simulink library "lib_Convection_TurbFlatPlatePowLawTempVary"  (R2015a)
settings: Solver=ode45  StartTime=0.0  StopTime=10.0  RelTol=1e-3
settings Model: Creator=jlkratz  LastModifiedBy=jlkratz

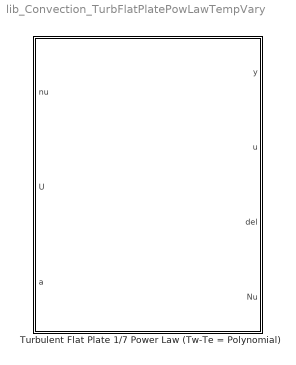
== system lib_Convection_TurbFlatPlatePowLawTempVary ==
  Turbulent Flat Plate 1/7 Power Law (Tw-Te = Polynomial) : Subsystem  mask(TSAT: Turbulent Flat Plate 1/7 Power Law (Tw-Te = Polynomial)){Pr_M=1, x_M=[0.05:0.05:5], n_M=50, BN_M=double(gcb)}
      mask prompts: Pr_M "Pr_M - Prandtl number"; x_M "x_M - Locations along the surface to compute the boundary layer for [mx1]"; n_M "n_M - Number of elements in the boundary layer"; BN_M "BN_M - Block name"
      mask help:
      | The block employs the 1/7 Power Law for incompressible turbulent flow over a flat plat with varying wall temperature (Tw) and or free-stream temperature (Te). The variation in temperature is assumed to be represented by a polynomial:
      |
      | Tw - Te = a0 + a1*x + a2*x^2 + ... + aN*x^N
      |
      | The 1/7 Power Law assumes the mean velocity (u) in the boundary layer and wall temperature minus the mean temperature (T) in the boundary layer vary with y^(1/7) where y is the distance from the surface of the wall. Temperature variations are accounted for using the method of indicial solutions based on the principle of superposition which is applicable give the thermal-energy equation is linear.
      |
      | See the block help menu for more details.
      mask init:
      | %Error/Warning Checking --------------------------------------------------%
      | 
      | %---- Pr_M ----%
      | %Scalar?
      | if isscalar(Pr_M) == 0
      |     Pr_M = 1;
      |     fprintf('Warning in %s: Pr_M must be a scalar. Pr_M has been set equal to 1 for computations.\n',char(BN_M));
      | end
      | %Real?
      | if isreal(Pr_M) == 0
      |     Pr_M = real(Pr_M);
      |     fprintf('Warning in %s: Pr_M must be a real. Pr_M has been set equal to real part of the entered value for computations.\n',char(BN_M));
      | end
      | %Finite?
      | if isfinite(Pr_M) == 0
      |     Pr_M = 1;
      |     fprintf('Warning in %s: Pr_M must be a finite. Pr_M has been set equal to 1 for computations.\n',char(BN_M));
      | end
      | %greater than 0
      | if Pr_M <= 0
      |     Pr_M = 0.01;
      |     fprintf('Warning in %s: Pr_M must be positive. Pr_M has been set equal to 0.01 for computations.\n',char(BN_M));
      | end
      | %Between 0.01 and 40000
      | if Pr_M < 0.01 || Pr_M > 40000
      |     fprintf('Warning in %s: Pr_M is outside of recommended range of Prandtl numbers (0.01 < Pr < 40000). Results could be erroneous.\n',char(BN_M));
      | end
      | %---- x_M ----%
      | %Not empty?
      | if isempty(x_M) == 1
      |     x_M = [0.1 0.5 1];
      |     fprintf('Warning in %s: x_M cannot be empty. x_M has been set to [0.1 0.5 1] for computations.\n',char(BN_M));
      | end
      | %1-D array?
      | if min(size(x_M)) ~= 1 || length(size(x_M)) > 2
      |     x_M = [0.1 0.5 1];
      |     fprintf('Warning in %s: x_M must be a 1-D array. x_M has been set to [0.1 0.5 1] for computations.\n',char(BN_M));
      | end
      | %Real?
      | if min(isreal(x_M)) == 0
      |     x_M = real(x_M);
      |     fprintf('Warning in %s: x_M must have all real elements. x_M has been set equal to the real parts of the entered values for computations.\n',char(BN_M));
      | end
      | %Finite?
      | if min(isfinite(x_M)) == 0
      |     x_M = [0.1 0.5 1];
      |     fprintf('Warning in %s: x_M must have all finite elements. x_M has been set equal to [0.1 0.5 1] for computations.\n',char(BN_M));
      | end
      | %Greater than 0?
      | if min(x_M) <= 0
      |     x_M = [0.1 0.5 1];
      |     fprintf('Warning in %s: x_M must have all elements that are greater than 0. x_M has been set equal to [0.1 0.5 1] for computations.\n',char(BN_M));
      | end
      | %Monotonically Increasing?
      | if max(size(x_M)) > 1
      |     if min(diff(x_M)) <= 0
      |         x_M = unique(sort(x_M));
      |         fprintf('Warning in %s: x_M must be a monotonically increasing array. x_M has been put in ascending order with redundant elements removed for computations\n',char(BN_M));
      |     end
      | end
      | %---- n_M ----%
      | %Scalar?
      | if isscalar(n_M) == 0
      |     n_M = 10;
      |     fprintf('Warning in %s: n_M must be a scalar. n_M has been set equal to 10 for computations.\n',char(BN_M));
      | end
      | %Real?
      | if isreal(n_M) == 0
      |     n_M = real(n_M);
      |     fprintf('Warning in %s: n_M must be a real. n_M has been set equal to real part of the entered value for computations.\n',char(BN_M));
      | end
      | %Finite?
      | if isfinite(n_M) == 0
      |     n_M = 10;
      |     fprintf('Warning in %s: n_M must be a finite. n_M has been set equal to 10 for computations.\n',char(BN_M));
      | end
      | %Integer?
      | if rem(n_M,1) > 0
      |     n_M = round(n_M);
      |     fprintf('Warning in %s: n_M must be an integer. n_M has been rounded to the closest integer.\n',char(BN_M));
      | end
      | %Greater than 1?
      | if n_M <= 1
      |     n_M = 2;
      |     fprintf('Warning in %s: n_M must be 2 or greater. n_M has been set equal to 2 for computations.\n',char(BN_M));
      | end
      mask Help: web(which('Convection_TSAT_TurbBLPowerLawTempVary.html'),'-helpbrowser')

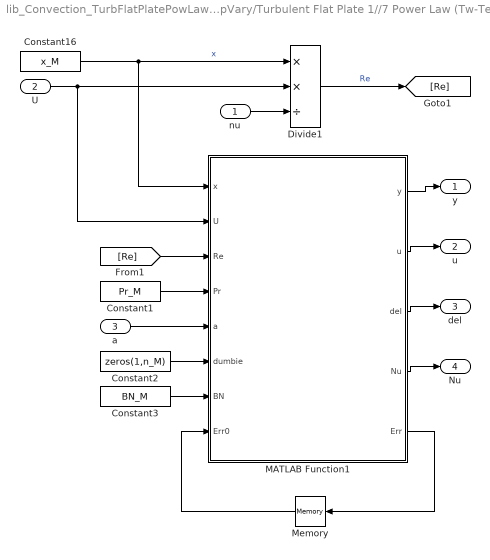
== system lib_Convection_TurbFlatPlatePowLawTempVary/Turbulent Flat Plate 1//7 Power Law (Tw-Te = Polynomial) ==
  nu : Inport
  U : Inport  Port=2
  a : Inport  Port=3
  Constant1 : Constant  Value=Pr_M
  Constant16 : Constant  Value=x_M
  Constant2 : Constant  Value=zeros(1,n_M)
  Constant3 : Constant  Value=BN_M
  Divide1 : Product  Inputs=**/
  MATLAB Function1 : MATLAB Function  TreatAsAtomicUnit=on
  Memory : Memory  X0=zeros(1,14)
  y : Outport
  u : Outport  Port=2
  del : Outport  Port=3
  Nu : Outport  Port=4
  wires:
  Constant2/1 -> MATLAB Function1/6(dumbie)
  Constant1/1 -> MATLAB Function1/4(Pr)
  U/1 -> Divide1/2, MATLAB Function1/2(U)
  a/1 -> MATLAB Function1/5(a)
  [Re] -> MATLAB Function1/3(Re)
  MATLAB Function1/3(del) -> del/1
  MATLAB Function1/4(Nu) -> Nu/1
  MATLAB Function1/1(y) -> y/1
  MATLAB Function1/2(u) -> u/1
  nu/1 -> Divide1/3
  Constant16/1 -> Divide1/1, MATLAB Function1/1(x)  "x"
  Divide1/1 -> [Re]  "Re"
  MATLAB Function1/5(Err) -> Memory/1
  Memory/1 -> MATLAB Function1/8(Err0)
  Constant3/1 -> MATLAB Function1/7(BN)

== matlab function lib_Convection_TurbFlatPlatePowLawTempVary/Turbulent Flat Plate 1//7 Power Law (Tw-Te = Polynomial)/MATLAB Function1 ==
  data: x input; U input; Re input; Pr input; a input; y output; u output; dumbie input; BN input; del output; Nu output; Err0 input; Err output
function [y, u, del, Nu, Err] = BoundaryLayerCalcs(x,U,Re,Pr,a,dumbie,BN,Err0)
%#codegen

%Description
% This function block computes dimensional quantities and forms the outputs

%Inputs:
% x - spatial variable along the surface [mx1]
% U - free-stream velocity [mx1]
% Re - Reynolds number [mx1]
% Pr - Prandtl number [1x1]
% a - array with polynomial coefficients for Tw-Te [px1]

%Outputs:
% y - dimensional y-coordinates for the velocity profile [nxm]
% U - velocity profile U(x,y) [nxm]
% del - hydrodynamic boundary layer thickness, del(x) [mx1]
% Nu - Nusselt number, Nu(x)[mx1]

%Error/Warning Checks ----------------------------------------------------%

Err = Err0;
ErrNum = 1;
%---- Re ----%
%Not empty?
if isempty(Re) == 1 &&  Err(ErrNum) == 0
    Err(ErrNum) = 1;
    fprintf('Warning in %s: Re is an empty array. It is suggested you check nu and x_M for sources of the error.\n',char(BN));
end
ErrNum = ErrNum + 1;
%1D array the length of x?
if (min(size(Re)) > 1 || length(size(Re)) > 2) && Err(ErrNum) == 0
    Err(ErrNum) = 1;
    fprintf('Warning in %s: Re must be a 1-D array. It is suggested you check nu and x_M for sources of the error.\n',char(BN));
end
ErrNum = ErrNum + 1;
%Real?
if min(isreal(Re)) < 1 && Err(ErrNum) == 0
    Err(ErrNum) = 1;
    fprintf('Warning in %s: Re must have all real elements. It is suggested you check nu and x_M for sources of the error.\n',char(BN));
end
ErrNum = ErrNum + 1;
%Finite?
if min(isfinite(Re)) < 1 && Err(ErrNum) == 0
    Err(ErrNum) = 1;
    fprintf('Warning in %s: Re must have all finite elements. It is suggested you check nu and x_M for sources of the error.\n',char(BN));
end
ErrNum = ErrNum + 1;
%Positive?
if min(Re) <= 0 && Err(ErrNum) == 0
    Err(ErrNum) = 1;
    fprintf('Warning in %s: Re must be great than 0. It is suggested you check nu and x_M for sources of the error.\n',char(BN));
end
ErrNum = ErrNum + 1;
%---- U ----%
%Not empty?
if isempty(U) == 1 &&  Err(ErrNum) == 0
    Err(ErrNum) = 1;
    fprintf('Warning in %s: U is an empty array.\n',char(BN));
end
ErrNum = ErrNum + 1;
%1D array the length of x?
if (min(size(U)) > 1 || length(size(U)) > 2) && Err(ErrNum) == 0
    Err(ErrNum) = 1;
    fprintf('Warning in %s: U must be a 1-D array.\n',char(BN));
end
ErrNum = ErrNum + 1;
%Real?
if min(isreal(U)) < 1 && Err(ErrNum) == 0
    Err(ErrNum) = 1;
    fprintf('Warning in %s: U must have all real elements.\n',char(BN));
end
ErrNum = ErrNum + 1;
%Finite?
if min(isfinite(U)) < 1 && Err(ErrNum) == 0
    Err(ErrNum) = 1;
    fprintf('Warning in %s: U must have all finite elements.\n',char(BN));
end
ErrNum = ErrNum + 1;
%Positive?
if min(U) <= 0 && Err(ErrNum) == 0
    Err(ErrNum) = 1;
    fprintf('Warning in %s: U must be great than 0.\n',char(BN));
end
ErrNum = ErrNum + 1;
%---- a ----%
%Not empty?
if isempty(a) == 1 && Err(ErrNum) == 0
    Err(ErrNum) = 1;
    fprintf('Warning in %s: a is empty.\n',char(BN));
end
ErrNum = ErrNum + 1;
%1D array > 1 element
if (length(size(a)) > 2 || min(size(a)) ~= 1) && length(a) < 2 && Err(ErrNum) == 0
    Err(ErrNum) = 1;
    fprintf('Warning in %s: a must be a 1D array with at least 2 elements.\n',char(BN));
end
ErrNum = ErrNum + 1;
%Real?
if min(isreal(a)) < 1 && Err(ErrNum) == 0
    Err(ErrNum) = 1;
    fprintf('Warning in %s: a must have all real elements.\n',char(BN));
end
ErrNum = ErrNum + 1;
%Finite?
if min(isfinite(a)) < 1 && Err(ErrNum) == 0
    Err(ErrNum) = 1;
    fprintf('Warning in %s: a must have all finitie elements.\n',char(BN));
end

%Initialize Outputs ------------------------------------------------------%

y = zeros(length(dumbie),length(x));
u = zeros(length(dumbie),length(x));
del = zeros(1,length(x));
Nu = zeros(1,length(x));

%Calculations ------------------------------------------------------------%

for j = 1:length(x)
    del(j) = 0.16*x(j)/Re(j)^(1/7);
end
y(1,:) = zeros(1,length(x));
for i = 2:length(dumbie)
    for j = 1:length(x)
        dy = del(j)/(length(dumbie)-1);
        y(i,j) = y(i-1,j) + dy;
        u(i,j) = U*(y(i,j)/del(j))^(1/7);
    end
end

St_ratio = zeros(1,length(x));
for j = 1:length(x)
    SUM = 0;
    for i = 2:length(a)
        SUM = SUM + (10/9)*(i-1)*a(i)*x(j)^(i-1)*(gamma(10*(i-1)/9)*gamma(8/9)/(gamma(10*(i-1)/9 + 8/9)));
    end
    TwmTe = 0;
    for i = 1:length(a)
        TwmTe = TwmTe + a(i)*x(j)^(i-1);
    end
    St_ratio(j) = (a(1) + SUM)/TwmTe;
    Cf = 0.455/(log(0.06*Re(j)))^2;
    St_dT = (Cf/2)/(1 + 13*(Pr^(2/3) - 1)*(Cf/2));
    St = St_dT*St_ratio(j);
    Nu(j) = St*Re(j)*Pr;
end
